simulink library "Feeder1_lib"  (Simulink 8.1)
settings: Solver=ode45  StartTime=0.0  StopTime=10.0  RelTol=1e-3
values from neighbouring files (symbols this model uses):
  Ts = 100E-6    (= 0.0001)    [BANSHEE_init.m]
undefined symbols (not defined in the file or in its folder): cable_spec, Left, type, V
libraries: breaker_lib x15, cables_lib x11, transformer_lib x7, ssn_lib x6, Load_lib x5, artemis x3, rtlab x2
settings Model: Creator=re25624  LastModifiedBy=re25624

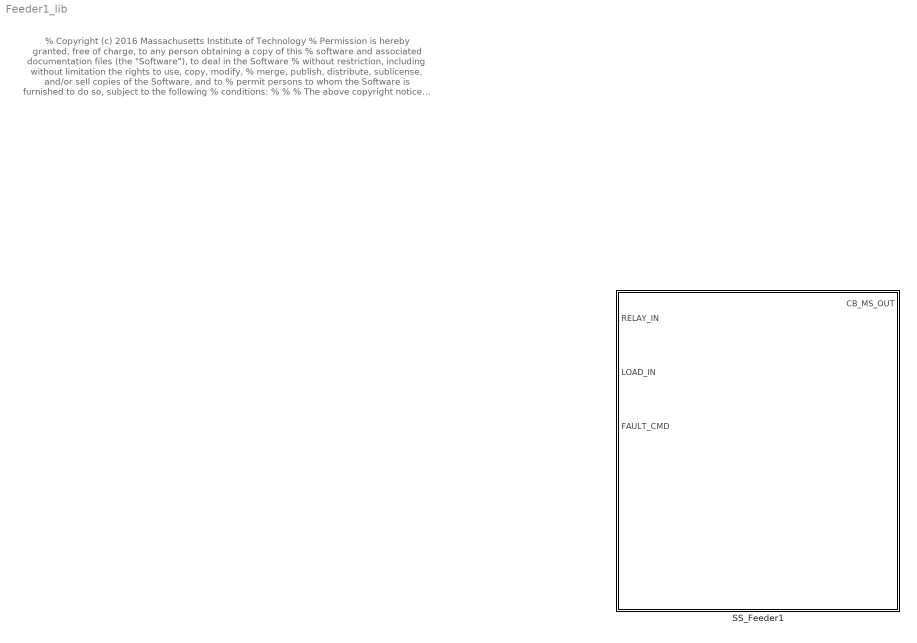
== system Feeder1_lib ==
  note: % Copyright (c) 2016 Massachusetts Institute of Technology
      | % Permission is hereby granted, free of charge, to any person obtaining a copy of this
      | % software and associated documentation files (the "Software"), to deal in the Software
      | % without restriction, including without limitation the rights to use, copy, modify,
      | % merge, publish, distribute, sublicense, and/or sell copies of the Software, and to
      | % permit persons to whom the Software is furnished to do so, subject to the following
      | % conditions:
      | %
      | %
      | % The above copyright notice and this permission notice shall be included in
      | % all copies or substantial portions of the Software.
      | %
      | % THE SOFTWARE IS PROVIDED "AS IS", WITHOUT WARRANTY OF ANY KIND, EXPRESS OR IMPLIED,
      | % INCLUDING BUT NOT LIMITED TO THE WARRANTIES OF MERCHANTABILITY, FITNESS FOR A
      | % PARTICULAR PURPOSE AND NONINFRINGEMENT. IN NO EVENT SHALL THE AUTHORS OR COPYRIGHT
      | % HOLDERS BE LIABLE FOR ANY CLAIM, DAMAGES OR OTHER LIABILITY, WHETHER IN AN ACTION
      | % OF CONTRACT, TORT OR OTHERWISE, ARISING FROM, OUT OF OR IN CONNECTION WITH THE
      | % SOFTWARE OR THE USE OR OTHER DEALINGS IN THE SOFTWARE.
      | %
      | %
      | %%
  SS_Feeder1 : Subsystem

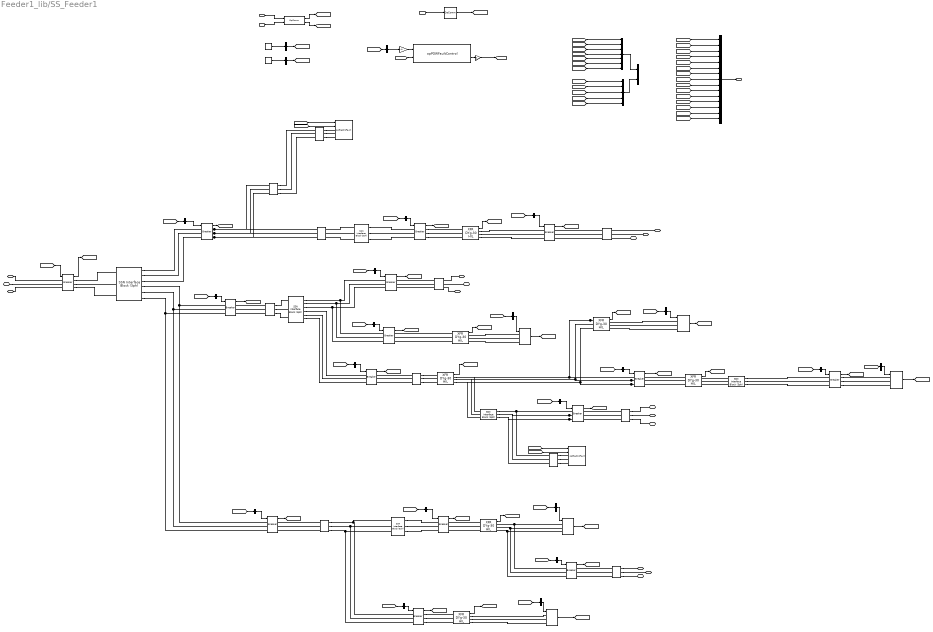
== system Feeder1_lib/SS_Feeder1 ==
  note: Point-on-wave synchronisation voltage (3-phase) in PU - Using 13.8 kV
  note: % Copyright (c) 2016 Massachusetts Institute of Technology
      | % Permission is hereby granted, free of charge, to any person obtaining a copy of this
      | % software and associated documentation files (the "Software"), to deal in the Software
      | % without restriction, including without limitation the rights to use, copy, modify,
      | % merge, publish, distribute, sublicense, and/or sell copies of the Software, and to
      | % permit persons to whom the Software is furnished to do so, subject to the following
      | % conditions:
      | %
      | %
      | % The above copyright notice and this permission notice shall be included in
      | % all copies or substantial portions of the Software.
      | %
      | % THE SOFTWARE IS PROVIDED "AS IS", WITHOUT WARRANTY OF ANY KIND, EXPRESS OR IMPLIED,
      | % INCLUDING BUT NOT LIMITED TO THE WARRANTIES OF MERCHANTABILITY, FITNESS FOR A
      | % PARTICULAR PURPOSE AND NONINFRINGEMENT. IN NO EVENT SHALL THE AUTHORS OR COPYRIGHT
      | % HOLDERS BE LIABLE FOR ANY CLAIM, DAMAGES OR OTHER LIABILITY, WHETHER IN AN ACTION
      | % OF CONTRACT, TORT OR OTHERWISE, ARISING FROM, OUT OF OR IN CONNECTION WITH THE
      | % SOFTWARE OR THE USE OR OTHER DEALINGS IN THE SOFTWARE.
      | %
      | %
      | %%
  note: connect to F3
  note: connect to F2
  note: connect to F2
  note: connect to F2
  note: Diesel
  note: motor
  RELAY_IN : Inport
  LOAD_IN : Inport  Port=2
  FAULT_CMD : Inport  Port=3
  2000 kVA4 : transformer_lib/XFR DYg-30 HIL  Rating=2000  Vp=4160  Vs=480  Z=5.75  XR=5.7
  2000 kVA5 : transformer_lib/XFR DYg-30 HIL  Rating=2000  Vp=4160  Vs=480  Z=5.75  XR=5.7
  2500 kVA : transformer_lib/XFR DYg-30 HIL  Rating=2500  Vp=13800  Vs=480  Z=5.75  XR=6.6
  2500 kVA2 : transformer_lib/XFR DYg-30 HIL  Rating=2500  Vp=13800  Vs=480  Z=5.56  XR=5.52
  3750 kVA1 : transformer_lib/XFR DYg-30 HIL  Rating=3750  Vp=13800  Vs=4160  Z=4.75  XR=11.4
  500 kVA2 : transformer_lib/XFR DYg-30 HIL  Rating=500  Vp=13800  Vs=480  Z=5  XR=4.9
  500 kVA3 : transformer_lib/XFR DYg-30 HIL  Rating=500  Vp=13800  Vs=208  Z=5  XR=4.9
  500kcmil_cable : cables_lib/500kcmil_cable  length=1  par_sets=1
  500kcmil_cable1 : cables_lib/500kcmil_cable  length=1  par_sets=1
  Bus Creator : BusCreator  Inputs=1
  Bus Creator1 : BusCreator  Inputs=1
  Bus Creator2 : BusCreator  Inputs=7
  Bus Creator3 : BusCreator  Inputs=5
  Bus Creator4 : BusCreator  Inputs=2
  Bus Creator5 : BusCreator  Inputs=15
  Bus Selector : BusSelector  OutputSignals=Vabc_bus
  Bus Selector1 : BusSelector  OutputSignals=F1_CB_12
  Bus Selector10 : BusSelector  OutputSignals=F1_CB_2
  Bus Selector11 : BusSelector  OutputSignals=F1_CB_1
  Bus Selector12 : BusSelector  OutputSignals=F1_CB_5
  Bus Selector13 : BusSelector  OutputSignals=F1_CB_3
  Bus Selector14 : BusSelector  OutputSignals=F1_CB_6
  Bus Selector15 : BusSelector  OutputSignals=F1_CB_7
  Bus Selector16 : BusSelector  OutputSignals=F1_CB_10
  Bus Selector17 : BusSelector  OutputSignals=F1_CB_11
  Bus Selector18 : BusSelector  OutputSignals=F1_CB_9
  Bus Selector19 : BusSelector  OutputSignals=F1_CB_14
  Bus Selector2 : BusSelector  OutputSignals=F1_CB_4
  Bus Selector3 : BusSelector  OutputSignals=I2
  Bus Selector4 : BusSelector  OutputSignals=C2
  Bus Selector5 : BusSelector  OutputSignals=P1
  Bus Selector6 : BusSelector  OutputSignals=C1
  Bus Selector7 : BusSelector  OutputSignals=I1
  Bus Selector8 : BusSelector  OutputSignals=F1_CB_13
  Bus Selector9 : BusSelector  OutputSignals=F1_CB_8
  C101 : cables_lib/PI-Section  cable_spec=[cable_spec(13, :)]  line_length=1800  parallel_sets=1
  C102 : cables_lib/PI-Section  cable_spec=[cable_spec(13, :)]  line_length=5500  parallel_sets=1
  C103 : cables_lib/PI-Section  cable_spec=[cable_spec(11, :)]  line_length=1000  parallel_sets=1
  C104 : cables_lib/PI-Section  cable_spec=[cable_spec(13, :)]  line_length=3000  parallel_sets=1
  C105 : cables_lib/PI-Section  cable_spec=[cable_spec(13, :)]  line_length=3000  parallel_sets=1
  C106 : cables_lib/PI-Section  cable_spec=[cable_spec(13, :)]  line_length=1500  parallel_sets=1
  C107 : cables_lib/PI-Section  cable_spec=[cable_spec(6, :)]  line_length=2000  parallel_sets=2
  C108 : cables_lib/PI-Section  cable_spec=[cable_spec(6, :)]  line_length=1000  parallel_sets=2
  C109 : cables_lib/PI-Section  cable_spec=[cable_spec(6, :)]  line_length=2000  parallel_sets=2
  CB closed : Constant
  CB open : Constant  Value=0
  Critical_1 : Load_lib/Dynamic_Load  V=460  Ts=Ts
  Critical_2 : Load_lib/Dynamic_Load  V=460  Ts=Ts
  F1_CB_{1..14} (14 alike) : breaker_lib/Breaker  Ts=Ts
  F1_PCC : breaker_lib/Breaker  Ts=Ts
  Interruptible_1 : Load_lib/Dynamic_Load  V=460  Ts=Ts
  Interruptible_2 : Load_lib/Dynamic_Load  V=208  Ts=Ts
  OpComm1 : rtlab/OpComm  nbport=2  groupe_acq=1  subsys_rate=0  st=0  Synchronization=on  Interpolation=on  Threshold=1.0  Missed_Data=off  Sim_Time=off  Samples=off  dynSigOut=off  from_console=0  warning_done=off  writeOpCommFile=off  Offset=off
  OpComm2 : rtlab/OpComm  nbport=1  groupe_acq=1  subsys_rate=0  st=0  Synchronization=on  Interpolation=on  Threshold=1.0  Missed_Data=off  Sim_Time=off  Samples=off  dynSigOut=off  from_console=1  warning_done=off  writeOpCommFile=off  Offset=off
  Priority_1 : Load_lib/Dynamic_Load  V=460  Ts=Ts
  SSN Interface Block (3ph) : ssn_lib/SSN Interface Block (3ph)  nb_phase=3  nb_port=3  p1_type=V-type(Left)  p2_type=V-type (Right)  p3_type=V-type (Right)  p4_type=V-type (Right)  p5_type=V-type(Left)  p6_type=V-type(Left)  p7_type=V-type(Left)  p8_type=V-type(Left)  p9_type=V-type(Left)  p10_type=V-type(Left)  p11_type=V-type(Left)  p12_type=V-type(Left)  p13_type=V-type(Left)  p14_type=V-type(Left)  p15_type=V-type(Left)  p16_type=V-type(Left)  I_port_shunt_resistance=1e9
  SSN Interface Block (3ph)1 : ssn_lib/SSN Interface Block (3ph)  nb_phase=3  nb_port=3  p1_type=V-type(Left)  p2_type=V-type (Right)  p3_type=V-type (Right)  p4_type=V-type(Left)  p5_type=V-type(Left)  p6_type=V-type(Left)  p7_type=V-type(Left)  p8_type=V-type(Left)  p9_type=V-type(Left)  p10_type=V-type(Left)  p11_type=V-type(Left)  p12_type=V-type(Left)  p13_type=V-type(Left)  p14_type=V-type(Left)  p15_type=V-type(Left)  p16_type=V-type(Left)  I_port_shunt_resistance=1e9
  SSN Interface Block (3ph){2..4,12} (4 alike) : ssn_lib/SSN Interface Block (3ph)  nb_phase=3  nb_port=2  p1_type=V-type(Left)  p2_type=V-type (Right)  p3_type=V-type(Left)  p4_type=V-type(Left)  p5_type=V-type(Left)  p6_type=V-type(Left)  p7_type=V-type(Left)  p8_type=V-type(Left)  p9_type=V-type(Left)  p10_type=V-type(Left)  p11_type=V-type(Left)  p12_type=V-type(Left)  p13_type=V-type(Left)  p14_type=V-type(Left)  p15_type=V-type(Left)  p16_type=V-type(Left)  I_port_shunt_resistance=1e9
  a : Gain  Gain=1/(13800*sqrt(2/3))
  opElectricFault : artemis/Tools /POW faults/opElectricFault  FaultLocation=location 2  FaultResistance=0.0001  GroundResistance=0.0001  InitialStates=[0 0 0]  SnubberResistance=1e6  SnubberCapacitance=inf
  opElectricFault1 : artemis/Tools /POW faults/opElectricFault  FaultLocation=location 3  FaultResistance=0.0001  GroundResistance=0.0001  InitialStates=[0 0 0]  SnubberResistance=1e6  SnubberCapacitance=inf
  opPOWFaultControl1 : artemis/Tools /POW faults/opPOWFaultControl  Ts=Ts  usePLL=off  Fgrid=60  PLL_k=[180 3200 1]  vol_sel=1: rising zero-corssing  SyncPhase_menu=A  T_acq=0.8
  triggerFAULT : Gain
  A_PCC : PMIOPort  Port=1  Side=Left
  B_PCC : PMIOPort  Port=2  Side=Left
  C_PCC : PMIOPort  Port=3  Side=Left
  A_CB_8 : PMIOPort  Port=4  Side=Right
  B_CB_8 : PMIOPort  Port=5  Side=Right
  C_CB_8 : PMIOPort  Port=6  Side=Right
  A_CB_11 : PMIOPort  Port=7  Side=Right
  B_CB_11 : PMIOPort  Port=8  Side=Right
  C_CB_11 : PMIOPort  Port=9  Side=Right
  A_CB_9 : PMIOPort  Port=10  Side=Right
  B_CB_9 : PMIOPort  Port=11  Side=Right
  C_CB_9 : PMIOPort  Port=12  Side=Right
  A_CB_13 : PMIOPort  Port=13  Side=Right
  B_CB_13 : PMIOPort  Port=14  Side=Right
  C_CB_13 : PMIOPort  Port=15  Side=Right
  CB_MS_OUT : Outport
  wires:
  [trigger] -> opElectricFault1/1
  [fault_cmd] -> opElectricFault1/2
  [trigger] -> opElectricFault/1
  [fault_cmd] -> opElectricFault/2
  FAULT_CMD/1 -> OpComm2/1
  OpComm2/1 -> [fault_cmd]
  a/1 -> opPOWFaultControl1/1
  Bus Selector/1 -> a/1  "<Vabc_bus>"
  [F1_PCC] -> Bus Selector/1
  triggerFAULT/1 -> [trigger]  "triggerFAULTsig"
  opPOWFaultControl1/2 -> triggerFAULT/1
  [fault_cmd] -> opPOWFaultControl1/2
  [F1_CB_14] -> Bus Creator5/14  "F1_CB_14"
  [F1_PCC] -> Bus Creator5/15  "F1_PCC"
  Bus Selector19/1 -> F1_CB_14/1  "<F1_CB_14>"
  [RELAY_IN] -> Bus Selector19/1
  F1_CB_14/1 -> [F1_CB_14]
  Bus Selector2/1 -> F1_CB_4/1  "<F1_CB_4>"
  [RELAY_IN] -> Bus Selector2/1
  F1_CB_4/1 -> [F1_CB_4]
  F1_CB_2/1 -> [F1_CB_2]
  Bus Selector18/1 -> F1_CB_9/1  "<F1_CB_9>"
  Bus Selector12/1 -> F1_CB_5/1  "<F1_CB_5>"
  Bus Selector11/1 -> F1_CB_1/1  "<F1_CB_1>"
  Bus Selector17/1 -> F1_CB_11/1  "<F1_CB_11>"
  Bus Selector16/1 -> F1_CB_10/1  "<F1_CB_10>"
  Bus Selector10/1 -> F1_CB_2/1  "<F1_CB_2>"
  Bus Selector14/1 -> F1_CB_6/1  "<F1_CB_6>"
  Bus Selector15/1 -> F1_CB_7/1  "<F1_CB_7>"
  Bus Selector9/1 -> F1_CB_8/1  "<F1_CB_8>"
  Bus Selector8/1 -> F1_CB_13/1  "<F1_CB_13>"
  Bus Selector1/1 -> F1_CB_12/1  "<F1_CB_12>"
  [RELAY_IN] -> Bus Selector18/1
  [RELAY_IN] -> Bus Selector17/1
  [RELAY_IN] -> Bus Selector16/1
  [RELAY_IN] -> Bus Selector15/1
  [RELAY_IN] -> Bus Selector14/1
  [RELAY_IN] -> Bus Selector12/1
  [RELAY_IN] -> Bus Selector11/1
  [RELAY_IN] -> Bus Selector10/1
  [RELAY_IN] -> Bus Selector9/1
  [RELAY_IN] -> Bus Selector8/1
  [RELAY_IN] -> Bus Selector1/1
  [RELAY_IN] -> Bus Selector13/1
  Bus Selector13/1 -> F1_CB_3/1  "<F1_CB_3>"
  Bus Creator5/1 -> CB_MS_OUT/1
  OpComm1/2 -> [RELAY_IN]
  RELAY_IN/1 -> OpComm1/2
  [F1_CB_2] -> Bus Creator5/2  "F1_CB_2"
  [F1_CB_3] -> Bus Creator5/3  "F1_CB_3"
  [F1_CB_4] -> Bus Creator5/4  "F1_CB_4"
  [F1_CB_5] -> Bus Creator5/5  "F1_CB_5"
  [F1_CB_6] -> Bus Creator5/6  "F1_CB_6"
  [F1_CB_7] -> Bus Creator5/7  "F1_CB_7"
  [F1_CB_8] -> Bus Creator5/8  "F1_CB_8"
  [F1_CB_9] -> Bus Creator5/9  "F1_CB_9"
  [F1_CB_10] -> Bus Creator5/10  "F1_CB_10"
  [F1_CB_11] -> Bus Creator5/11  "F1_CB_11"
  [F1_CB_12] -> Bus Creator5/12  "F1_CB_12"
  [F1_CB_13] -> Bus Creator5/13  "F1_CB_13"
  [F1_CB_1] -> Bus Creator5/1  "F1_CB_1"
  F1_CB_11/1 -> [F1_CB_11]
  F1_CB_10/1 -> [F1_CB_10]
  F1_CB_13/1 -> [F1_CB_13]
  F1_CB_12/1 -> [F1_CB_12]
  F1_CB_8/1 -> [F1_CB_8]
  F1_CB_7/1 -> [F1_CB_7]
  F1_CB_6/1 -> [F1_CB_6]
  F1_CB_9/1 -> [F1_CB_9]
  F1_CB_5/1 -> [F1_CB_5]
  F1_CB_1/1 -> [F1_CB_1]
  F1_CB_3/1 -> [F1_CB_3]
  [LOAD_I1] -> Bus Creator3/3  "F1_I1"
  [LOAD_C2] -> Bus Creator3/2  "F1_C2"
  [LOAD_P1] -> Bus Creator3/5  "F1_P1"
  [LOAD_I2] -> Bus Creator3/4  "F1_I2"
  [XFM_F1_2] -> Bus Creator2/2  "F1_X2"
  [XFM_F1_3] -> Bus Creator2/3  "F1_X3"
  [XFM_F1_4] -> Bus Creator2/4  "F1_X4"
  [XFM_F1_5] -> Bus Creator2/5  "F1_X5"
  [XFM_F1_6] -> Bus Creator2/6  "F1_X6"
  [XFM_F1_7] -> Bus Creator2/7  "F1_X7"
  Bus Creator3/1 -> Bus Creator4/2  "LOAD"
  Bus Creator2/1 -> Bus Creator4/1  "XFR"
  [LOAD_C1] -> Bus Creator3/1  "F1_C1"
  [XFM_F1_1] -> Bus Creator2/1  "F1_X1"
  Interruptible_1/1 -> [LOAD_I1]
  Critical_1/1 -> [LOAD_C1]
  Priority_1/1 -> [LOAD_P1]
  Critical_2/1 -> [LOAD_C2]
  Interruptible_2/1 -> [LOAD_I2]
  2500 kVA/1 -> [XFM_F1_7]
  500 kVA3/1 -> [XFM_F1_6]
  2000 kVA4/1 -> [XFM_F1_5]
  2000 kVA5/1 -> [XFM_F1_4]
  3750 kVA1/1 -> [XFM_F1_3]
  2500 kVA2/1 -> [XFM_F1_2]
  500 kVA2/1 -> [XFM_F1_1]
  Bus Selector7/1 -> Interruptible_1/1  "<I1>"
  Bus Selector6/1 -> Critical_1/1  "<C1>"
  Bus Selector5/1 -> Priority_1/1  "<P1>"
  Bus Selector4/1 -> Critical_2/1  "<C2>"
  Bus Selector3/1 -> Interruptible_2/1  "<I2>"
  [LOAD_IN] -> Bus Selector7/1
  [LOAD_IN] -> Bus Selector6/1
  [LOAD_IN] -> Bus Selector5/1
  [LOAD_IN] -> Bus Selector4/1
  [LOAD_IN] -> Bus Selector3/1
  OpComm1/1 -> [LOAD_IN]
  LOAD_IN/1 -> OpComm1/1
  CB open/1 -> Bus Creator1/1  "Logic_trip"
  Bus Creator1/1 -> [cb_o]
  CB closed/1 -> Bus Creator/1  "Logic_trip"
  Bus Creator/1 -> [cb_c]
  F1_PCC/1 -> [F1_PCC]
  [cb_c] -> F1_PCC/1
  connections:
  500kcmil_cable1/RConn2 -- opElectricFault1/LConn2
  500kcmil_cable1/RConn1 -- opElectricFault1/LConn1
  500kcmil_cable1/RConn3 -- opElectricFault1/LConn3
  C103/RConn3 -- 500kcmil_cable/LConn3
  C103/RConn2 -- 500kcmil_cable/LConn2
  C103/RConn1 -- 500kcmil_cable/LConn1
  500kcmil_cable/RConn2 -- opElectricFault/LConn2
  500kcmil_cable/RConn1 -- opElectricFault/LConn1
  500kcmil_cable/RConn3 -- opElectricFault/LConn3
  SSN Interface Block (3ph)4/RConn1 -- F1_CB_14/LConn1
  SSN Interface Block (3ph)4/RConn3 -- F1_CB_14/LConn3
  SSN Interface Block (3ph)4/RConn2 -- F1_CB_14/LConn2
  SSN Interface Block (3ph)4/LConn1 -- 2000 kVA5/RConn1
  SSN Interface Block (3ph)4/LConn3 -- 2000 kVA5/RConn3
  SSN Interface Block (3ph)4/LConn2 -- 2000 kVA5/RConn2
  500 kVA2/RConn3 -- Interruptible_1/LConn3
  500 kVA2/RConn1 -- Interruptible_1/LConn1
  500 kVA2/RConn2 -- Interruptible_1/LConn2
  C106/RConn1 -- 3750 kVA1/LConn1
  C106/RConn3 -- 3750 kVA1/LConn3
  C106/RConn2 -- 3750 kVA1/LConn2
  SSN Interface Block (3ph)1/RConn5 -- F1_CB_6/LConn2
  SSN Interface Block (3ph)1/RConn4 -- F1_CB_6/LConn1
  SSN Interface Block (3ph)1/RConn6 -- F1_CB_6/LConn3
  F1_CB_7/LConn3 -- SSN Interface Block (3ph)1/RConn3 -- F1_CB_8/LConn3
  F1_CB_7/LConn2 -- SSN Interface Block (3ph)1/RConn2 -- F1_CB_8/LConn2
  F1_CB_7/LConn1 -- SSN Interface Block (3ph)1/RConn1 -- F1_CB_8/LConn1
  2000 kVA4/LConn1 -- 3750 kVA1/RConn1 -- SSN Interface Block (3ph)12/LConn1 -- F1_CB_10/LConn1
  F1_CB_11/LConn2 -- SSN Interface Block (3ph)12/RConn2 -- 500kcmil_cable1/LConn2
  F1_CB_10/LConn3 -- 3750 kVA1/RConn3 -- SSN Interface Block (3ph)12/LConn3 -- 2000 kVA4/LConn3
  SSN Interface Block (3ph)3/RConn3 -- F1_CB_12/LConn3
  SSN Interface Block (3ph)3/RConn1 -- F1_CB_12/LConn1
  SSN Interface Block (3ph)3/RConn2 -- F1_CB_12/LConn2
  SSN Interface Block (3ph)3/LConn1 -- C104/RConn1
  SSN Interface Block (3ph)3/LConn3 -- C104/RConn3
  SSN Interface Block (3ph)3/LConn2 -- C104/RConn2
  B_CB_8/RConn1 -- C105/RConn2
  C_CB_8/RConn1 -- C105/RConn3
  A_CB_8/RConn1 -- C105/RConn1
  C105/LConn1 -- F1_CB_8/RConn1
  C105/LConn3 -- F1_CB_8/RConn3
  C105/LConn2 -- F1_CB_8/RConn2
  A_CB_13/RConn1 -- C109/RConn1
  B_CB_13/RConn1 -- C109/RConn2
  C_CB_13/RConn1 -- C109/RConn3
  C109/LConn2 -- F1_CB_13/RConn2
  C109/LConn3 -- F1_CB_13/RConn3
  C109/LConn1 -- F1_CB_13/RConn1
  F1_PCC/RConn3 -- SSN Interface Block (3ph)/LConn3
  F1_PCC/RConn1 -- SSN Interface Block (3ph)/LConn1
  F1_PCC/RConn2 -- SSN Interface Block (3ph)/LConn2
  SSN Interface Block (3ph)/RConn3 -- F1_CB_3/LConn3
  SSN Interface Block (3ph)/RConn2 -- F1_CB_3/LConn2
  SSN Interface Block (3ph)/RConn1 -- F1_CB_3/LConn1
  SSN Interface Block (3ph)2/RConn3 -- F1_CB_5/LConn3
  SSN Interface Block (3ph)2/RConn1 -- F1_CB_5/LConn1
  SSN Interface Block (3ph)2/RConn2 -- F1_CB_5/LConn2
  F1_CB_14/RConn3 -- Priority_1/LConn3
  F1_CB_14/RConn2 -- Priority_1/LConn2
  F1_CB_14/RConn1 -- Priority_1/LConn1
  F1_CB_4/RConn2 -- 500 kVA2/LConn2
  F1_CB_4/RConn3 -- 500 kVA2/LConn3
  F1_CB_4/RConn1 -- 500 kVA2/LConn1
  C107/RConn2 -- B_CB_11/RConn1
  C107/RConn3 -- C_CB_11/RConn1
  C107/RConn1 -- A_CB_11/RConn1
  C108/RConn2 -- B_CB_9/RConn1
  C108/RConn1 -- A_CB_9/RConn1
  C108/RConn3 -- C_CB_9/RConn1
  SSN Interface Block (3ph)12/RConn1 -- F1_CB_11/LConn1 -- 500kcmil_cable1/LConn1
  F1_CB_10/LConn2 -- 3750 kVA1/RConn2 -- SSN Interface Block (3ph)12/LConn2 -- 2000 kVA4/LConn2
  F1_CB_11/LConn3 -- SSN Interface Block (3ph)12/RConn3 -- 500kcmil_cable1/LConn3
  Interruptible_2/LConn1 -- 500 kVA3/RConn1
  Critical_1/LConn3 -- F1_CB_9/LConn3 -- 2500 kVA2/RConn3
  SSN Interface Block (3ph)2/LConn1 -- C101/RConn1 -- F1_CB_4/LConn1
  2500 kVA/RConn3 -- F1_CB_13/LConn3
  C_PCC/RConn1 -- F1_PCC/LConn3
  Interruptible_2/LConn2 -- 500 kVA3/RConn2
  SSN Interface Block (3ph)2/LConn2 -- C101/RConn2 -- F1_CB_4/LConn2
  500 kVA3/LConn2 -- F1_CB_7/RConn2
  500 kVA3/LConn1 -- F1_CB_7/RConn1
  2500 kVA/RConn1 -- F1_CB_13/LConn1
  C108/LConn3 -- F1_CB_9/RConn3
  F1_CB_3/RConn3 -- C103/LConn3 -- C104/LConn3
  C101/LConn3 -- F1_CB_1/RConn3
  C108/LConn2 -- F1_CB_9/RConn2
  C108/LConn1 -- F1_CB_9/RConn1
  F1_CB_3/RConn1 -- C103/LConn1 -- C104/LConn1
  2000 kVA5/LConn3 -- F1_CB_10/RConn3
  Critical_2/LConn2 -- 2000 kVA4/RConn2
  C101/LConn2 -- F1_CB_1/RConn2
  500 kVA3/LConn3 -- F1_CB_7/RConn3
  F1_CB_12/RConn3 -- 2500 kVA/LConn3
  C101/LConn1 -- F1_CB_1/RConn1
  Critical_2/LConn3 -- 2000 kVA4/RConn3
  F1_CB_12/RConn2 -- 2500 kVA/LConn2
  2000 kVA5/LConn2 -- F1_CB_10/RConn2
  Interruptible_2/LConn3 -- 500 kVA3/RConn3
  C106/LConn3 -- F1_CB_6/RConn3
  F1_CB_3/RConn2 -- C103/LConn2 -- C104/LConn2
  B_PCC/RConn1 -- F1_PCC/LConn2
  2500 kVA2/LConn1 -- F1_CB_5/RConn1
  2000 kVA5/LConn1 -- F1_CB_10/RConn1
  A_PCC/RConn1 -- F1_PCC/LConn1
  C106/LConn2 -- F1_CB_6/RConn2
  SSN Interface Block (3ph)/RConn4 -- F1_CB_2/LConn1 -- F1_CB_1/LConn1
  SSN Interface Block (3ph)/RConn5 -- F1_CB_2/LConn2 -- F1_CB_1/LConn2
  SSN Interface Block (3ph)/RConn6 -- F1_CB_2/LConn3 -- F1_CB_1/LConn3
  F1_CB_12/RConn1 -- 2500 kVA/LConn1
  SSN Interface Block (3ph)2/LConn3 -- C101/RConn3 -- F1_CB_4/LConn3
  Critical_1/LConn1 -- F1_CB_9/LConn1 -- 2500 kVA2/RConn1
  C102/LConn1 -- F1_CB_2/RConn1
  C102/LConn3 -- F1_CB_2/RConn3
  2500 kVA2/LConn2 -- F1_CB_5/RConn2
  C102/LConn2 -- F1_CB_2/RConn2
  2500 kVA2/LConn3 -- F1_CB_5/RConn3
  2500 kVA/RConn2 -- F1_CB_13/LConn2
  C106/LConn1 -- F1_CB_6/RConn1
  Critical_1/LConn2 -- F1_CB_9/LConn2 -- 2500 kVA2/RConn2
  Critical_2/LConn1 -- 2000 kVA4/RConn1
  C102/RConn2 -- SSN Interface Block (3ph)1/LConn2
  C102/RConn3 -- SSN Interface Block (3ph)1/LConn3
  C102/RConn1 -- SSN Interface Block (3ph)1/LConn1
  C107/LConn1 -- F1_CB_11/RConn1
  C107/LConn2 -- F1_CB_11/RConn2
  C107/LConn3 -- F1_CB_11/RConn3
